simulink model "f14_airframe"  (R2026b)
settings: Solver=VariableStepAuto  MaxStep=0.1  EnableMultiTasking=on
undefined symbols (not defined in the file): Md, Mq, Mw, Uo, Zd
libraries: simulink x2
settings Model: DataDictionary=system_model.sldd  ModifiedByFormat=The MathWorks Inc.  Creator=The MathWorks, Inc.  LastModifiedBy=The MathWorks Inc.
settings DataIOCC: LimitDataPoints=on  ReturnWorkspaceOutputs=off  SaveFormat=Array  SaveOutput=off  SaveTime=off  SignalLogging=off  SignalLoggingName=f14_airframe
settings OptimizationCC: DefaultParameterBehavior=Inlined  LifeSpan=inf  MemsetInitFltsAndDblsToZero=off
settings DebuggingCC: AllowSymbolicDim=off  ArithmeticOperatorsInVariantConditions=warning  FcnCallInpInsideContextMsg=warning  MergeDetectMultiDrivingBlocksExec=none  MultiTaskCondExecSysMsg=none  MultiTaskDSMMsg=warning  PregeneratedLibrarySubsystemCodeDiagnostic=none  SFExecutionAtInitializationDiag=none  SFNoUnconditionalDefaultTransitionDiag=warning  SFUnexpectedBacktrackingDiag=warning  SaveWithParameterizedLinksMsg=none  SignalResolutionControl=TryResolveAllWithWarning  SolverPrmCheckMsg=warning  StateNameClashWarn=warning  UnderspecifiedInitializationDetection=Classic
settings HardwareCC: ProdEndianess=Unspecified  ProdHWDeviceType=32-bit Generic  ProdIntDivRoundTo=Undefined  ProdLargestAtomicFloat=None
settings ModelReferenceCC: PropagateSignalLabelsOutOfModel=off
settings SFSimCC: CustomCodeUndefinedFunction=UseInterfaceOnly  SimUseLocalCustomCode=off
settings RTWCC: RTWUseLocalCustomCode=off
settings CodeAppCC: StateflowObjectComments=on
settings GRTTargetCC: CombineOutputUpdateFcns=off  GRTInterface=on  TargetFcnLib=ansi_tfl_tmw.mat  TargetLangStandard=C89/C90 (ANSI)
settings ConfigComp: CovExternalEMLEnable=off  CovSFcnEnable=off  CovSaveCumulativeToWorkspaceVar=on  CovSaveSingleToWorkspaceVar=on

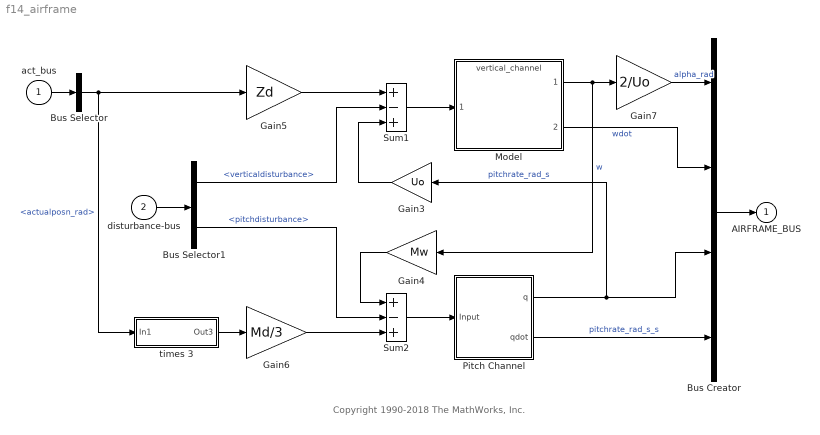
== system f14_airframe ==
  note: Copyright 1990-2018 The MathWorks, Inc.
  act_bus : Inport  OutDataTypeStr=Bus: ACT_BUS
  disturbance-bus : Inport  Port=2  OutDataTypeStr=Bus: DISTURB_BUS
  Bus Creator : BusCreator  Inputs='alpha_rad','wdot','pitchrate_rad_s','pitchrate_rad_s_s'  OutDataTypeStr=Bus: AIRFRAME_BUS
  Bus Selector : BusSelector  OutputSignals=actualposn_rad
  Bus Selector1 : BusSelector  OutputSignals=verticaldisturbance,pitchdisturbance
  Gain3 : Gain  Gain=Uo  SaturateOnIntegerOverflow=on  OutDataTypeStr=Inherit: Same as input  ParamDataTypeStr=Inherit: Same as input
  Gain4 : Gain  Gain=Mw  SaturateOnIntegerOverflow=on  OutDataTypeStr=Inherit: Same as input  ParamDataTypeStr=Inherit: Same as input
  Gain5 : Gain  Gain=Zd  SaturateOnIntegerOverflow=on  OutDataTypeStr=Inherit: Same as input  ParamDataTypeStr=Inherit: Same as input
  Gain6 : Gain  Gain=Md/3  SaturateOnIntegerOverflow=on  OutDataTypeStr=Inherit: Same as input  ParamDataTypeStr=Inherit: Same as input
  Gain7 : Gain  Gain=2/Uo  SaturateOnIntegerOverflow=on  OutDataTypeStr=Inherit: Same as input  ParamDataTypeStr=Inherit: Same as input
  Model : ModelReference  ModelNameDialog=vertical_channel  SimulationMode=Normal  ModelReferenceVersion=12.0
  Pitch Channel : Subsystem
  Sum1 : Sum  Inputs=+-+  InputSameDT=on  SaturateOnIntegerOverflow=on  OutDataTypeStr=Inherit: Same as first input
  Sum2 : Sum  Inputs=+-+  InputSameDT=on  SaturateOnIntegerOverflow=on  OutDataTypeStr=Inherit: Same as first input
  "times 3 " : Subsystem
  AIRFRAME_BUS : Outport  OutDataTypeStr=Bus: AIRFRAME_BUS  InitialOutput=0  VectorParamsAs1DForOutWhenUnconnected=off  BusOutputAsStruct=on
  wires:
  Gain4/1 -> Sum2/1
  Gain3/1 -> Sum1/3
  Gain7/1 -> Bus Creator/1  "alpha_rad"
  Bus Selector1/1 -> Sum1/2  "<verticaldisturbance>"
  Sum2/1 -> Pitch Channel/1(Input)
  Bus Selector1/2 -> Sum2/2  "<pitchdisturbance>"
  Gain5/1 -> Sum1/1
  Gain6/1 -> Sum2/3
  Sum1/1 -> Model/1
  Model/1 -> Gain7/1, Gain4/1  "w"
  Model/2 -> Bus Creator/2  "wdot"
  Pitch Channel/1(q) -> Gain3/1, Bus Creator/3  "pitchrate_rad_s"
  Pitch Channel/2(qdot) -> Bus Creator/4  "pitchrate_rad_s_s"
  act_bus/1 -> Bus Selector/1
  Bus Selector/1 -> "times 3 "/1(In1), Gain5/1  "<actualposn_rad>"
  Bus Creator/1 -> AIRFRAME_BUS/1
  disturbance-bus/1 -> Bus Selector1/1
  "times 3 "/1(Out3) -> Gain6/1

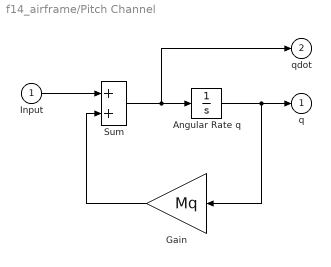
== system f14_airframe/Pitch Channel ==
  Input : Inport
  "Angular Rate q " : Integrator
  Gain : Gain  Gain=Mq  SaturateOnIntegerOverflow=on  OutDataTypeStr=Inherit: Same as input  ParamDataTypeStr=Inherit: Same as input
  Sum : Sum  InputSameDT=on  SaturateOnIntegerOverflow=on  OutDataTypeStr=Inherit: Same as first input
  q : Outport  VectorParamsAs1DForOutWhenUnconnected=off
  qdot : Outport  Port=2  VectorParamsAs1DForOutWhenUnconnected=off
  wires:
  Sum/1 -> qdot/1, "Angular Rate q "/1
  "Angular Rate q "/1 -> Gain/1, q/1
  Gain/1 -> Sum/2
  Input/1 -> Sum/1

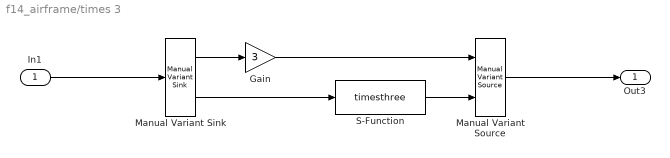
== system f14_airframe/times 3  ==
  In1 : Inport
  Gain : Gain  Gain=3
  Manual Variant Sink : simulink/Signal Routing/Manual Variant Sink  NumChoices=2  LabelModeActiveChoice=V_1
  Manual Variant Source : simulink/Signal Routing/Manual Variant Source  NumChoices=2  LabelModeActiveChoice=V_1
  S-Function : S-Function  FunctionName=timesthree  SFunctionDeploymentMode=off  EnableBusSupport=off
  Out3 : Outport  VectorParamsAs1DForOutWhenUnconnected=off
  wires:
  In1/1 -> Manual Variant Sink/1
  Manual Variant Sink/2 -> S-Function/1
  S-Function/1 -> Manual Variant Source/2
  Gain/1 -> Manual Variant Source/1
  Manual Variant Source/1 -> Out3/1
  Manual Variant Sink/1 -> Gain/1
